simulink model "SuddenChangeVel"  (R2017b)
settings: Solver=VariableStepAuto  StartTime=0.0  StopTime=4  RelTol=1e-3
settings Model: Creator=81068  LastModifiedBy=81068

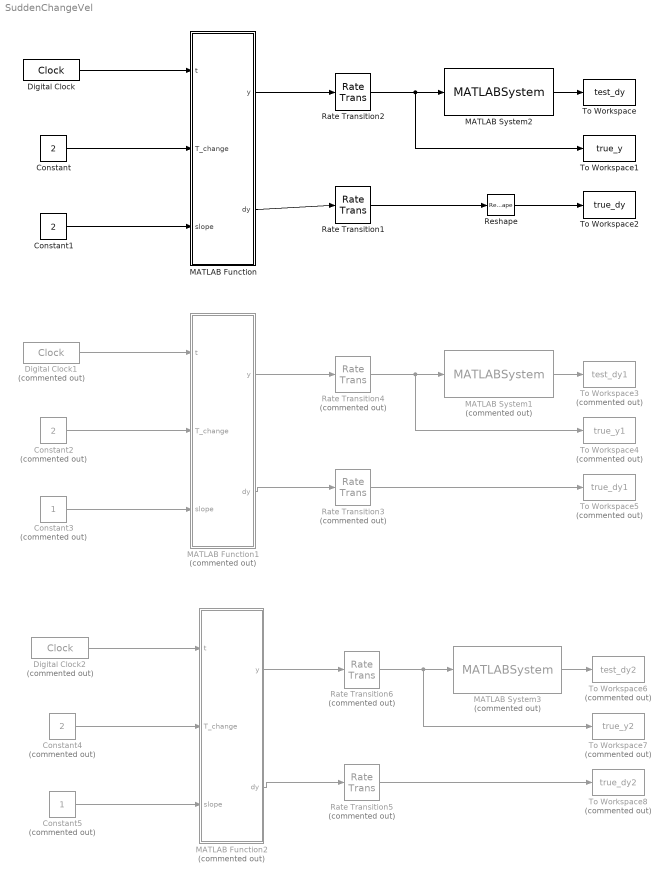
== system SuddenChangeVel ==
  Constant : Constant  Value=2
  Constant1 : Constant  Value=2
  Constant2 : Constant  Commented=on  Value=2
  Constant3 : Constant  Commented=on
  Constant4 : Constant  Commented=on  Value=2
  Constant5 : Constant  Commented=on
  Digital Clock : DigitalClock  SampleTime=1/2000
  Digital Clock1 : DigitalClock  Commented=on  SampleTime=1/2000
  Digital Clock2 : DigitalClock  Commented=on  SampleTime=1/2000
  MATLAB Function : MATLAB Function  TreatAsAtomicUnit=on
  MATLAB Function1 : MATLAB Function  Commented=on  TreatAsAtomicUnit=on
  MATLAB Function2 : MATLAB Function  Commented=on  TreatAsAtomicUnit=on
  MATLAB System1 : MATLABSystem  Commented=on  System=PolyRegressionFilter  sample_time=1/2000  history_length=3  dop=1  signal_dim=1  delay=0  SimulateUsing=Code generation
      mask Type: PolyRegressionFilter
      mask Display:
      | disp('PolyRegressionFilter');
      | port_label('input',1,'q');
      | port_label('output',1,'dq');
  MATLAB System2 : MATLABSystem  System=PolyRegressionFilter  sample_time=1/2000  history_length=3  dop=1  signal_dim=1  delay=0  SimulateUsing=Code generation
      mask Type: PolyRegressionFilter
      mask Display:
      | disp('PolyRegressionFilter');
      | port_label('input',1,'q');
      | port_label('output',1,'dq');
  MATLAB System3 : MATLABSystem  Commented=on  System=PolyRegressionFilter  sample_time=1/2000  history_length=3  dop=1  signal_dim=1  delay=0  SimulateUsing=Code generation
      mask Type: PolyRegressionFilter
      mask Display:
      | disp('PolyRegressionFilter');
      | port_label('input',1,'q');
      | port_label('output',1,'dq');
  Rate Transition1 : RateTransition  OutPortSampleTime=sample_time
  Rate Transition2 : RateTransition  OutPortSampleTime=sample_time
  Rate Transition{3..6} (4 alike) : RateTransition  Commented=on  OutPortSampleTime=sample_time
  Reshape : Reshape  OutputDimensionality=Column vector (2-D)
  To Workspace : ToWorkspace  VariableName=test_dy  SaveFormat=Timeseries  SampleTime=-1
  To Workspace1 : ToWorkspace  VariableName=true_y  SaveFormat=Timeseries  SampleTime=-1
  To Workspace2 : ToWorkspace  VariableName=true_dy  SaveFormat=Timeseries  SampleTime=-1
  To Workspace3 : ToWorkspace  Commented=on  VariableName=test_dy1  SaveFormat=Timeseries  SampleTime=-1
  To Workspace4 : ToWorkspace  Commented=on  VariableName=true_y1  SaveFormat=Timeseries  SampleTime=-1
  To Workspace5 : ToWorkspace  Commented=on  VariableName=true_dy1  SaveFormat=Timeseries  SampleTime=-1
  To Workspace6 : ToWorkspace  Commented=on  VariableName=test_dy2  SaveFormat=Timeseries  SampleTime=-1
  To Workspace7 : ToWorkspace  Commented=on  VariableName=true_y2  SaveFormat=Timeseries  SampleTime=-1
  To Workspace8 : ToWorkspace  Commented=on  VariableName=true_dy2  SaveFormat=Timeseries  SampleTime=-1
  wires:
  Digital Clock/1 -> MATLAB Function/1(t)
  MATLAB Function/1(y) -> Rate Transition2/1
  MATLAB System2/1 -> To Workspace/1
  Rate Transition2/1 -> To Workspace1/1, MATLAB System2/1
  MATLAB Function/2(dy) -> Rate Transition1/1
  Rate Transition1/1 -> Reshape/1
  Constant1/1 -> MATLAB Function/3(slope)
  Constant/1 -> MATLAB Function/2(T_change)
  Constant2/1 -> MATLAB Function1/2(T_change)
  Rate Transition3/1 -> To Workspace5/1
  MATLAB Function1/2(dy) -> Rate Transition3/1
  Constant3/1 -> MATLAB Function1/3(slope)
  Digital Clock1/1 -> MATLAB Function1/1(t)
  Rate Transition4/1 -> To Workspace4/1, MATLAB System1/1
  MATLAB Function1/1(y) -> Rate Transition4/1
  MATLAB System1/1 -> To Workspace3/1
  Constant4/1 -> MATLAB Function2/2(T_change)
  Rate Transition5/1 -> To Workspace8/1
  MATLAB Function2/2(dy) -> Rate Transition5/1
  Constant5/1 -> MATLAB Function2/3(slope)
  Digital Clock2/1 -> MATLAB Function2/1(t)
  Rate Transition6/1 -> To Workspace7/1, MATLAB System3/1
  MATLAB Function2/1(y) -> Rate Transition6/1
  MATLAB System3/1 -> To Workspace6/1
  Reshape/1 -> To Workspace2/1

== matlab function SuddenChangeVel/MATLAB Function1 ==
  data: t input; y output; dy output; T_change input; slope input
function [y,dy] = position_signal(t,T_change,slope)%,T_change,slope)
if t<T_change
    y = slope*t;
    dy = slope;
else
    y = slope*T_change;
    dy = 0;
end

== matlab function SuddenChangeVel/MATLAB Function ==
  data: t input; y output; dy output; T_change input; slope input
function [y,dy] = position_signal(t,T_change,slope)%,T_change,slope)
if t<T_change
    y = slope*t;
    dy = slope;
else
    y = slope*T_change;
    dy = 0;
end

== matlab function SuddenChangeVel/MATLAB Function2 ==
  data: t input; y output; dy output; T_change input; slope input
function [y,dy] = position_signal(t,T_change,slope)%,T_change,slope)
if t<T_change
    y = slope*t;
    dy = slope;
else
    y = slope*T_change;
    dy = 0;
end
